simulink model "host_uart_wifi"  (Simulink 7.3)
settings: Solver=VariableStepDiscrete  StartTime=0.0  StopTime=inf  RelTol=1e-3
libraries: waijung_socket_lib x1
settings Model: Creator=Krisada  LastModifiedBy=Krisada

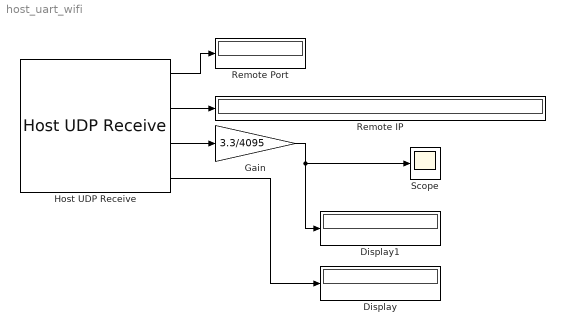
== system host_uart_wifi ==
  Display : Display
      settings: Format=hex (Stored Integer)
  Display1 : Display
  Gain : Gain  Gain=3.3/4095  ParameterDataType=fixdt(1, 16)  ParameterScaling=2^0  OutDataType=fixdt(1, 16)  OutScaling=2^0
  Host UDP Receive : waijung_socket_lib/Host UDP Receive  Priority=1  conf=HostReceive  protocol=UDP  port=7  address=192.168.1.31  echo=off  transfer=Blocking  timeout=5  datasource=Ports  datatype=uint8  datacount=2  porttype_double=0  porttype_single=0  porttype_int8=0  porttype_uint8=0  porttype_int16=0  porttype_uint16=0  porttype_int32=0  porttype_uint32=2  portpinstr=0  sampletime=0.001  blockid=HostUDPReceive  inputporttype=[]  inputportwidth=[]  inputportlabel={}  outputporttype=[5,3,7,7]  outputportwidth=[1,4,]  outputportlabel={'Remote Port','Remote IP(1:4)','uint32 D0','uint32 D1'}  compat=0  optionstring="[\"UDP\",\"7\",\"192\",\"168\",\"1\",\"21\",\"Non-blocking\",\"PortData\",\"uint8_t\",\"2\",\"Send\",\"off\"]"  options=[7,2,1,5000,0]
  Remote IP : Display
  Remote Port : Display
  Scope : Scope
      settings: YMin=3.291  YMax=3.301
  wires:
  Host UDP Receive/1 -> Remote Port/1
  Host UDP Receive/2 -> Remote IP/1
  Gain/1 -> Display1/1, Scope/1
  Host UDP Receive/3 -> Gain/1
  Host UDP Receive/4 -> Display/1
